simulink model "model"  (R2015a)
settings: Solver=ode45  StartTime=0.0  StopTime=40  MaxStep=0.01  RelTol=1e-3
values from neighbouring files (symbols this model uses):
  A = double((A + A') /2 > 0)    [init.m]    (also in init_consensus.m = ones(n) - eye(n); init_trust_consensus.m = ones(n) - eye(n))
  adapt = 1    [init.m]    (also in init_model.m; init_mussels.m; init_mussels_2.m; init_mussels_konfiguracija_blizu.m)
  c = [ 0   0.2   0   0   0 ... (first row only)    [init.m]    (also in init_mussels.m = zeros(n,n); init_mussels_2.m; init_mussels_konfiguracija_blizu.m = [ 0   0.2   0.7   0.8   0.9; init_mussels_konfiguracija_daleko.m = [ 0   0.2   0.7   0.8   0.9)
  K = 0.02    [init.m]    (also in init_model.m; init_mussels.m; init_mussels_2.m; init_mussels_konfiguracija_blizu.m)
  n = input(prompt)    [init.m]    (also in init_consensus.m = 4; init_consensus_15.m = 15; init_mussels.m = 5; init_mussels_2.m = 5)
  sigma_0 = [ 0    0.7   0    0    0 ... (first row only)    [init.m]    (also in init_model.m = zeros(M,M); init_mussels.m = zeros(n,n); init_mussels_2.m; init_mussels_konfiguracija_blizu.m = [ 0    0.7   0.4    0.6    0.5)
  zeta_0 = zeros(n,n)    [init.m]    (also in init_model.m = zeros(M,M); init_mussels.m; init_mussels_2.m; init_mussels_konfiguracija_blizu.m)
settings Model: Creator=Marta_2805  LastModifiedBy=Tamara
settings SolverCC: AutoInsertRateTranBlk=on
settings DebuggingCC: UnderspecifiedInitializationDetection=Classic  MergeDetectMultiDrivingBlocksExec=none  SolverPrmCheckMsg=warning

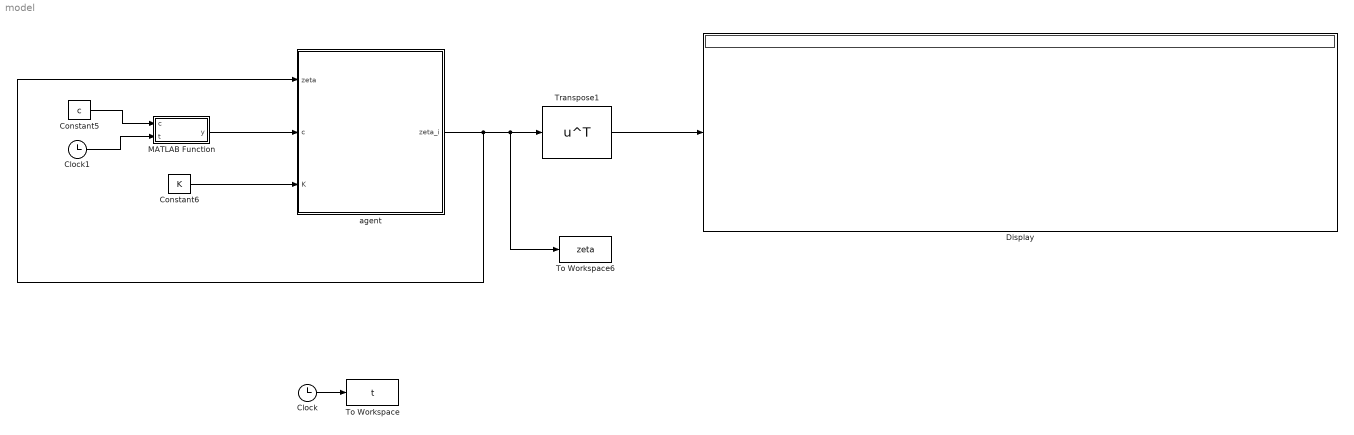
== system model ==
  Clock : Clock
  Clock1 : Clock
  Constant5 : Constant  Value=c
  Constant6 : Constant  Value=K
  Display : Display
  MATLAB Function : MATLAB Function  TreatAsAtomicUnit=on
  To Workspace : ToWorkspace  VariableName=t  SampleTime=-1
  To Workspace6 : ToWorkspace  VariableName=zeta  SampleTime=-1
  Transpose1 : Math  Operator=transpose  SaturateOnIntegerOverflow=on
  "agent " : Subsystem
  wires:
  Constant6/1 -> "agent "/3(K)
  MATLAB Function/1(y) -> "agent "/2(c)
  "agent "/1(zeta_i) -> "agent "/1(zeta), To Workspace6/1, Transpose1/1
  Transpose1/1 -> Display/1
  Clock/1 -> To Workspace/1
  Constant5/1 -> MATLAB Function/1(c)
  Clock1/1 -> MATLAB Function/2(t)

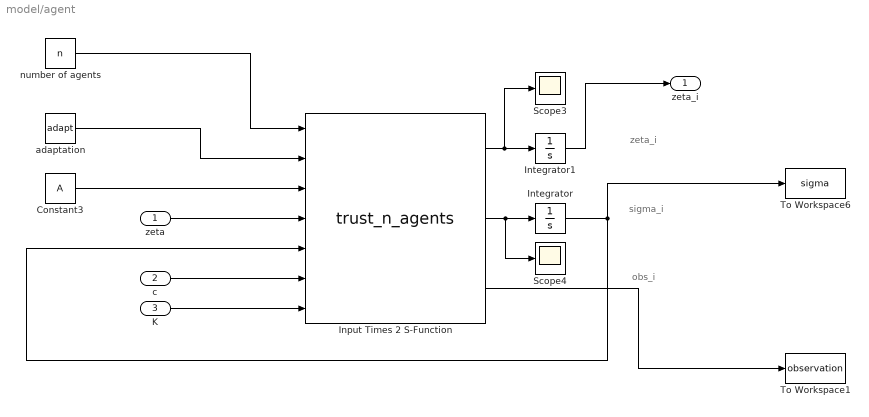
== system model/agent  ==
  note: obs_i
  note: sigma_i
  note: zeta_i
  zeta : Inport
  c : Inport  Port=2
  K : Inport  Port=3
  Constant3 : Constant  Value=A
  Input Times 2 S-Function : S-Function  FunctionName=trust_n_agents
  Integrator : Integrator  InitialCondition=sigma_0
  Integrator1 : Integrator  InitialCondition=zeta_0
  Scope3 : Scope
      settings: TimeRange=20  YMin=0.25  YMax=0.95  SaveName=ScopeData3
  Scope4 : Scope
      settings: TimeRange=20  YMin=0.25  YMax=0.95  SaveName=ScopeData4
  To Workspace1 : ToWorkspace  VariableName=observation  SampleTime=-1
  To Workspace6 : ToWorkspace  VariableName=sigma  SampleTime=-1
  adaptation : Constant  Value=adapt
  number of agents : Constant  Value=n
  zeta_i : Outport
  wires:
  Integrator/1 -> Input Times 2 S-Function/5, To Workspace6/1
  Integrator1/1 -> zeta_i/1
  c/1 -> Input Times 2 S-Function/6
  K/1 -> Input Times 2 S-Function/7
  Input Times 2 S-Function/2 -> Scope4/1, Integrator/1
  Input Times 2 S-Function/1 -> Scope3/1, Integrator1/1
  Input Times 2 S-Function/3 -> To Workspace1/1
  number of agents/1 -> Input Times 2 S-Function/1
  adaptation/1 -> Input Times 2 S-Function/2
  Constant3/1 -> Input Times 2 S-Function/3
  zeta/1 -> Input Times 2 S-Function/4

== matlab function model/MATLAB Function ==
  data: c input; y output; t input
function y = fcn(c, t)
%#codegen
if t > 25
    c(:,1) = c(:,1);
%    c(:,13) = c(:,13) / 5; 
%    c(:,13) = c(:,13) / 7;
%    c(:,3) = c(:,3) * 2;
end
y = c;
